simulink model "HTHmodel"  (R2025a)
settings: Solver=VariableStepAuto  StartTime=0.0  StopTime=259200  FixedStep=1  MaxStep=10  RelTol=1e-3  AbsTol=1e-6
PreLoadFcn:
  | HTHmodel_ini
model workspace (MATLAB code in the model file):
  | % load initial conditions and physical properties from file
  | 
  | HTHmodel_ini
values from neighbouring files (symbols this model uses):
  c = 4005.4    [HTHmodel_ini.m]
  cost = 0.09/3.6e6    (= 2.5e-08)    [HTHmodel_ini.m]
  M = (lenHouse*widHouse*htHouse+tan(pitRoof)*widHouse*lenHouse)*densAir    [HTHmodel_ini.m]
  Mdot = 1    [HTHmodel_ini.m]
  Req = RWall*RWindow/(RWall + RWindow)    [HTHmodel_ini.m]
  THeater = 50    [HTHmodel_ini.m]
  TinIC = 10    [HTHmodel_ini.m]
Description:
  | DT model for a residential scale rooftop PV system.
  | 
  | FMI.V2 tool has been utilized for cross-platform model exchange interoperability.
  | 
  | The simulation is offline and conducted for three days.
settings Model: ExtModeTrigDuration=100  Creator=The MathWorks, Inc.  LastModifiedBy=DR53SF
settings SolverCC: AutoScaleAbsTol=off  AlgebraicLoopSolver=TrustRegion
settings DataIOCC: ExternalInput=[]  InitialState=[]
settings OptimizationCC: BlockReduction=off  BooleanDataType=off  ReuseModelBlockBuffer=off  ExpressionDepthLimit=2147483647.0  InitFltsAndDblsToZero=on  LifeSpan=inf  BufferReusableBoundary=off
settings DebuggingCC: SaveWithParameterizedLinksMsg=none  UnderspecifiedInitializationDetection=Classic  MergeDetectMultiDrivingBlocksExec=none  SignalResolutionControl=TryResolveAllWithWarning  MultiTaskDSMMsg=warning  MultiTaskCondExecSysMsg=none  IntegerOverflowMsg=none  FcnCallInpInsideContextMsg=warning  UnconnectedInputMsg=warning  UnconnectedOutputMsg=warning  UnconnectedLineMsg=warning  BusObjectLabelMismatch=none  StateNameClashWarn=warning  SFUnexpectedBacktrackingDiag=warning  SFNoUnconditionalDefaultTransitionDiag=warning  SFExecutionAtInitializationDiag=none  IntegerSaturationMsg=none  ArithmeticOperatorsInVariantConditions=warning
settings HardwareCC: ProdBitPerPointer=32.0  ProdBitPerSizeT=32.0  ProdBitPerPtrDiffT=32.0  ProdLargestAtomicFloat=None  ProdIntDivRoundTo=Undefined  ProdEndianess=Unspecified  ProdWordSize=32.0  ProdHWDeviceType=32-bit Generic  TargetUnknown=on
settings ModelReferenceCC: EnableRefExpFcnMdlSchedulingChecks=on  PropagateSignalLabelsOutOfModel=off
settings SFSimCC: SimUseLocalCustomCode=off  CustomCodeUndefinedFunction=UseInterfaceOnly
settings RTWCC: RTWUseLocalCustomCode=off  GPUComputeCapability=3.5
settings CodeAppCC: StateflowObjectComments=on
settings GRTTargetCC: TargetFcnLib=ansi_tfl_tmw.mat  TargetLangStandard=C89/C90 (ANSI)  CombineOutputUpdateFcns=off  GRTInterface=on
settings ConfigComp: CovMetricSettings=dw  CovSaveCumulativeToWorkspaceVar=on  CovSaveSingleToWorkspaceVar=on  CovExternalEMLEnable=off

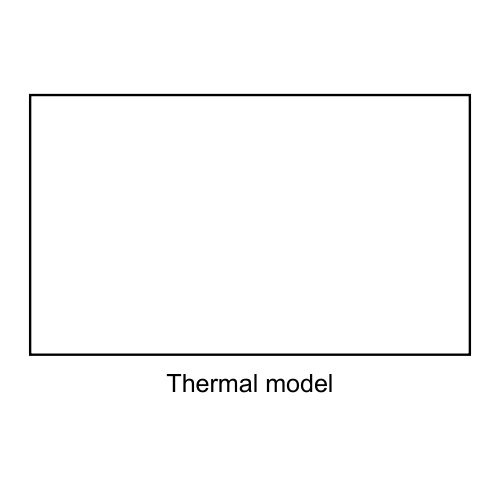
[thumbnail: Simulink's stored preview of the top-level diagram]
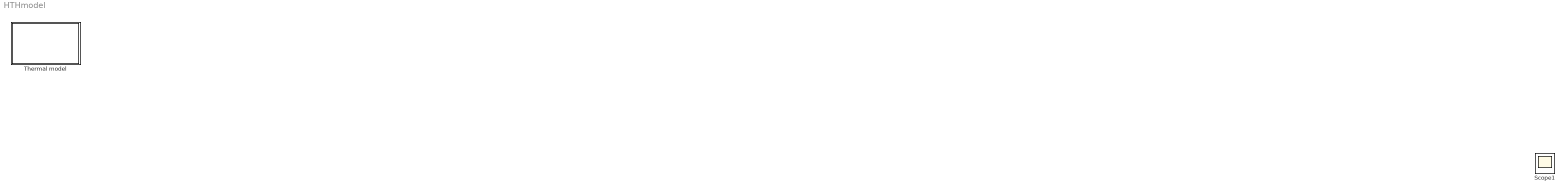
== system HTHmodel ==
  Thermal model : Subsystem
  Scope1 : Scope
      settings: ActiveDisplayYMinimum=-0.125  ActiveDisplayYMaximum=1.125

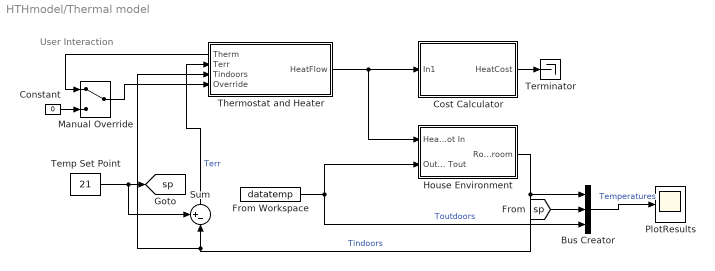
== system HTHmodel/Thermal model ==
  note: User Interaction
  Bus Creator : BusCreator  Inputs=3
  Constant : Constant  Value=0
  Cost Calculator : Subsystem
  From Workspace : FromWorkspace  VariableName=datatemp
  House Environment : Subsystem
  Manual Override : ManualSwitch
  PlotResults : Scope
      settings: ActiveDisplayYMinimum=-3.15766  ActiveDisplayYMaximum=28.41891  YLabel=HeatCost (in $)
  Sum : Sum  Inputs=+-|  InputSameDT=on  SaturateOnIntegerOverflow=on  OutDataTypeStr=Inherit: Same as first input
  Temp Set Point : Constant  Value=21
  Terminator : Terminator
  Thermostat and Heater : Subsystem
      settings: PortSchema="{\"entries\":[{\"content\":{\"sides\":[{\"content\":{\"connectorIds\":[\"Out2\",\"In1\",\"In2\",\"In3\"]},\"type\":\"ConnectorPlacement.EquallySpacedRectSide\",\"uuid\":\"4ecfb517-8ebb-45dc-a4b9-a5ae67d58104\"},{\"content\":{\"connectorIds\":[\"Out1\"],\"side\":\"RIGHT\"},\"type\":\"ConnectorPlacement.EquallySpacedRectSide\",\"uuid\":\"09859c0f-ddcc-4dd5-9669-1a419b60c2c9\"},{\"content\":{\"side\":\"TOP\"},\"type\":\"ConnectorPlacement.EquallySpacedRectSide\",\"uuid\":\"889fdd7c-aa0e-4a01-99e5-4dbd6aa0cac4\"}]},\"type\":\"ConnectorPlacement.EquallySpacedConnector\",\"uuid\":\"15962a41-2ec0-4669-962c-97a1a36d0320\"}],\"packageUris\":[\"http://schema.mathworks.com/mf0/Connector/R2020b\"],\"version\":\"1.0\"}"
  tag scope: sp=global
  wires:
  From Workspace/1 -> House Environment/2(Outdoor Temp Tout), Bus Creator/3  "Toutdoors"
  Temp Set Point/1 -> Sum/1, [sp]
  House Environment/1(Room Temp Troom) -> Sum/2, Thermostat and Heater/2(Tindoors), Bus Creator/1  "Tindoors"
  Bus Creator/1 -> PlotResults/1  "Temperatures"
  [sp] -> Bus Creator/2
  Thermostat and Heater/1(HeatFlow) -> House Environment/1(Heater QDot In), Cost Calculator/1(In1)
  Sum/1 -> Thermostat and Heater/1(Terr)  "Terr"
  Manual Override/1 -> Thermostat and Heater/3(Override)
  Thermostat and Heater/2(Therm) -> Manual Override/1
  Constant/1 -> Manual Override/2
  Cost Calculator/1(HeatCost) -> Terminator/1

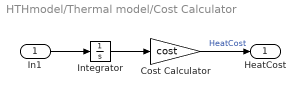
== system HTHmodel/Thermal model/Cost Calculator ==
  In1 : Inport
  Cost Calculator : Gain  Gain=cost  SaturateOnIntegerOverflow=on  OutDataTypeStr=Inherit: Same as input  ParamDataTypeStr=Inherit: Same as input
  Integrator : Integrator
  HeatCost : Outport
  wires:
  Integrator/1 -> Cost Calculator/1
  Cost Calculator/1 -> HeatCost/1  "HeatCost"
  In1/1 -> Integrator/1

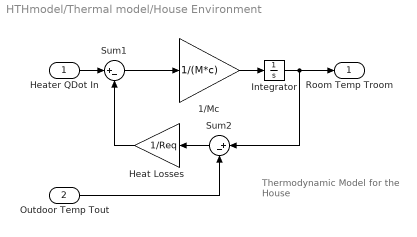
== system HTHmodel/Thermal model/House Environment ==
  note: Thermodynamic Model
      | for the House
  Heater QDot In : Inport
  Outdoor Temp Tout : Inport  Port=2
  1/Mc : Gain  Gain=1/(M*c)  SaturateOnIntegerOverflow=on  OutDataTypeStr=Inherit: Same as input  ParamDataTypeStr=Inherit: Same as input
  Heat Losses : Gain  Gain=1/Req  SaturateOnIntegerOverflow=on  OutDataTypeStr=Inherit: Same as input  ParamDataTypeStr=Inherit: Same as input
  Integrator : Integrator  InitialCondition=TinIC
  Sum1 : Sum  Inputs=|+-  InputSameDT=on  SaturateOnIntegerOverflow=on  OutDataTypeStr=Inherit: Same as first input
  Sum2 : Sum  Inputs=|+-  InputSameDT=on  SaturateOnIntegerOverflow=on  OutDataTypeStr=Inherit: Same as first input
  Room Temp Troom : Outport  InitialOutput=0  VectorParamsAs1DForOutWhenUnconnected=off
  wires:
  Outdoor Temp Tout/1 -> Sum2/2
  Heater QDot In/1 -> Sum1/1
  Sum1/1 -> 1/Mc/1
  Sum2/1 -> Heat Losses/1
  Heat Losses/1 -> Sum1/2
  1/Mc/1 -> Integrator/1
  Integrator/1 -> Sum2/1, Room Temp Troom/1

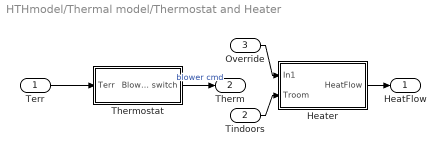
== system HTHmodel/Thermal model/Thermostat and Heater ==
  Terr : Inport
  Tindoors : Inport  Port=2
  Override : Inport  Port=3
  Heater : Subsystem
  Thermostat : Subsystem
  HeatFlow : Outport
  Therm : Outport  Port=2
  wires:
  Heater/1(HeatFlow) -> HeatFlow/1
  Thermostat/1(Blower switch) -> Therm/1  "blower cmd"
  Terr/1 -> Thermostat/1(Terr)
  Tindoors/1 -> Heater/2(Troom)
  Override/1 -> Heater/1(In1)

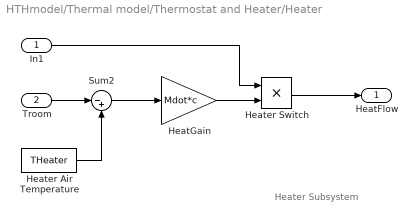
== system HTHmodel/Thermal model/Thermostat and Heater/Heater ==
  note: Heater Subsystem
  In1 : Inport
  Troom : Inport  Port=2
  HeatGain : Gain  Gain=Mdot*c
  Heater Air Temperature : Constant  Value=THeater
  Heater Switch : Product  RndMeth=Zero
  Sum2 : Sum  Inputs=|-+
  HeatFlow : Outport  VectorParamsAs1DForOutWhenUnconnected=off
  wires:
  Heater Air Temperature/1 -> Sum2/2
  Troom/1 -> Sum2/1
  Sum2/1 -> HeatGain/1
  HeatGain/1 -> Heater Switch/2
  Heater Switch/1 -> HeatFlow/1
  In1/1 -> Heater Switch/1

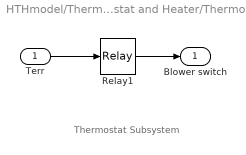
== system HTHmodel/Thermal model/Thermostat and Heater/Thermostat ==
  note: Thermostat Subsystem
  Terr : Inport
  Relay1 : Relay  OnSwitchValue=2  OffSwitchValue=-2
  Blower switch : Outport  InitialOutput=0  VectorParamsAs1DForOutWhenUnconnected=off
  wires:
  Terr/1 -> Relay1/1
  Relay1/1 -> Blower switch/1
